simulink model "schemat_lab7"  (R2020a)
settings: Solver=VariableStepAuto  StartTime=0.0  StopTime=10.0  RelTol=1e-3
values from neighbouring files (symbols this model uses):
  A = [(-a1/A1), (a1/A1); (a1/A2), ((-a1-a2)/A2)]    [gotowe2.m]    (also in lab7.m)
  B = [ (1/A1) ,    0   ;  0,        (1/A2)     ]    [gotowe2.m]    (also in lab7.m)
  C = [1,0;0,1]    [gotowe2.m]    (also in lab7.m)
  D = zeros(2)    [gotowe2.m]    (also in lab7.m)
  dfwe1 = 0    [gotowe2.m]    (also in lab7.m; lab8.m = 0.5)
  dfwe2 = 0.1*fwemax    (= 0.5)    [gotowe2.m]    (also in lab7.m = 0; lab8.m = 0)
  fwe1 = 1    [gotowe2.m]    (also in lab7.m = mfwe1(i)*fwemax; lab8.m = mfwe1(i)*fwemax)
  fwe2 = mfwe2*fwemax    (= 2.5)    [gotowe2.m]    (also in lab7.m = 1; lab8.m = 1)
  h = -(A^(-1))*B*u    [gotowe2.m]    (also in lab7.m)
settings Model: Creator=pc  LastModifiedBy=pc

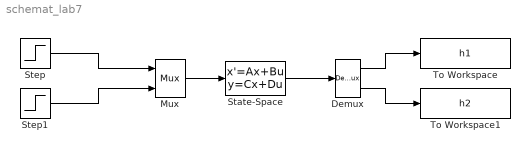
== system schemat_lab7 ==
  Demux : Demux  Outputs=2
  Mux : Mux  Inputs=2
  State-Space : StateSpace  A=A  B=B  C=C  D=D  InitialCondition=h
  Step : Step  Time=5  Before=fwe1  After=fwe1+dfwe1  SampleTime=0
  Step1 : Step  Time=5  Before=fwe2  After=fwe2+dfwe2  SampleTime=0
  To Workspace : ToWorkspace  VariableName=h1  SampleTime=-1
  To Workspace1 : ToWorkspace  VariableName=h2  SampleTime=-1
  wires:
  Step/1 -> Mux/1
  Step1/1 -> Mux/2
  Mux/1 -> State-Space/1
  State-Space/1 -> Demux/1
  Demux/1 -> To Workspace/1
  Demux/2 -> To Workspace1/1
